simulink model "Hybrid2_article_SVC_stage1"  (R2025a)
settings: Solver=FixedStepAuto  StartTime=0.0  StopTime=0.2  FixedStep=Ts  RelTol=1e-3
undefined symbols (not defined in the file or in its folder): closedLoop, controller, D1, D11, Delta, DiscIntNeverNeededParam, find_system, grid, level, protection, sensor, solarPanel, solarPlant, Ts
libraries: powerlib_extras x38, nesl_utility x29, spsSampleandHoldLib x24, spsThyristorLib x24, spsSeriesRLCBranchLib x23, simulink x22, fl_lib x18, ee_lib x12, spsEdgeDetectorLib x12, spsParallelRLCBranchLib x10, spsThreePhaseVIMeasurementLib x9, simulink_extras x8
(part 3 of 8)

== system Hybrid2_article_SVC_stage1/TSC4 ==
  note: Firing pulses
  note: TSC1
  P : Inport  PortDimensions=6
  Bus to Vector : BusToVector
  Cab : spsSeriesRLCBranchLib/Series RLC Branch  LConnTagsString=__new0  RConnTagsString=__new0  BranchType=RC  Resistance=Rseries  Inductance=1.0  SetiL0=off  InitialCurrent=0  Capacitance=Ccmt  Setx0=off  InitialVoltage=0  Measurements=Branch voltage and current
  Cbc : spsSeriesRLCBranchLib/Series RLC Branch  LConnTagsString=__new0  RConnTagsString=__new0  BranchType=RC  Resistance=Rseries  Inductance=1.0  SetiL0=off  InitialCurrent=0  Capacitance=Ccmt  Setx0=off  InitialVoltage=0  Measurements=None
  Cca : spsSeriesRLCBranchLib/Series RLC Branch  LConnTagsString=__new0  RConnTagsString=__new0  BranchType=RC  Resistance=Rseries  Inductance=1.0  SetiL0=off  InitialCurrent=0  Capacitance=Ccmt  Setx0=off  InitialVoltage=0  Measurements=None
  Demux : Demux  Outputs=6
      settings: DisplayOption=none
  Lab : spsParallelRLCBranchLib/Parallel RLC Branch  LConnTagsString=a  RConnTagsString=__new0  BranchType=RL  Resistance=Rparallel  Inductance=Lcmt  SetiL0=off  InitialCurrent=0  Capacitance=1.0  Setx0=off  InitialVoltage=0  Measurements=None
  Lbc : spsParallelRLCBranchLib/Parallel RLC Branch  LConnTagsString=a  RConnTagsString=__new0  BranchType=RL  Resistance=Rparallel  Inductance=Lcmt  SetiL0=off  InitialCurrent=0  Capacitance=1.0  Setx0=off  InitialVoltage=0  Measurements=None
  Lca : spsParallelRLCBranchLib/Parallel RLC Branch  LConnTagsString=a  RConnTagsString=__new0  BranchType=RL  Resistance=Rparallel  Inductance=Lcmt  SetiL0=off  InitialCurrent=0  Capacitance=1.0  Setx0=off  InitialVoltage=0  Measurements=None
  Selector6 : Selector  InputPortWidth=2  IndexOptions=Index vector (dialog)  Indices=2  OutputSizes=1
  ThAB+ : spsThyristorLib/Thyristor  Ron=Ron  Lon=0  Vf=Vf  IC=0  Rs=Rsnub  Cs=Csnub  Measurements=on
      settings: AttributesFormatString=\n
  ThAB- : spsThyristorLib/Thyristor  Ron=Ron  Lon=0  Vf=Vf  IC=0  Rs=inf  Cs=0  Measurements=off
      settings: AttributesFormatString=\n
  ThBC+ : spsThyristorLib/Thyristor  Ron=Ron  Lon=0  Vf=Vf  IC=0  Rs=Rsnub  Cs=Csnub  Measurements=off
      settings: AttributesFormatString=\n
  ThBC- : spsThyristorLib/Thyristor  Ron=Ron  Lon=0  Vf=Vf  IC=0  Rs=inf  Cs=0  Measurements=off
      settings: AttributesFormatString=\n
  ThCA+ : spsThyristorLib/Thyristor  Ron=Ron  Lon=0  Vf=Vf  IC=0  Rs=Rsnub  Cs=Csnub  Measurements=off
      settings: AttributesFormatString=\n
  ThCA- : spsThyristorLib/Thyristor  Ron=Ron  Lon=0  Vf=Vf  IC=0  Rs=inf  Cs=0  Measurements=off
      settings: AttributesFormatString=\n
  A : PMIOPort  Side=Left
  B : PMIOPort  Port=2  Side=Left
  C : PMIOPort  Port=3  Side=Left
  tag scope: Vth_TSC1ab=global
  wires:
  P/1 -> Demux/1
  [Ap] -> ThAB+/1
  Demux/1 -> [Ap]
  Demux/2 -> [Am]
  Demux/3 -> [Bp]
  Demux/4 -> [Bm]
  Demux/5 -> [Cp]
  [Am] -> ThAB-/1
  [Bp] -> ThBC+/1
  [Bm] -> ThBC-/1
  [Cp] -> ThCA+/1
  [Cm] -> ThCA-/1
  Demux/6 -> [Cm]
  ThAB+/1 -> Bus to Vector/1
  Selector6/1 -> [Vth_TSC1ab]
  Bus to Vector/1 -> Selector6/1
  connections:
  Lab/RConn1 -- Cab/LConn1
  Lab/LConn1 -- ThAB-/LConn1 -- ThAB+/RConn1
  Cca/RConn1 -- A/RConn1 -- ThAB+/LConn1 -- ThAB-/RConn1
  Lbc/LConn1 -- ThBC-/LConn1 -- ThBC+/RConn1
  Cab/RConn1 -- ThBC-/RConn1 -- ThBC+/LConn1 -- B/RConn1
  Lca/LConn1 -- ThCA-/LConn1 -- ThCA+/RConn1
  Cbc/RConn1 -- ThCA-/RConn1 -- ThCA+/LConn1 -- C/RConn1
  Lbc/RConn1 -- Cbc/LConn1
  Lca/RConn1 -- Cca/LConn1

== system Hybrid2_article_SVC_stage1/TSC5 ==
  note: Firing pulses
  P : Inport  PortDimensions=6
  Cab : spsSeriesRLCBranchLib/Series RLC Branch  LConnTagsString=__new0  RConnTagsString=__new0  BranchType=RC  Resistance=Rseries  Inductance=1.0  SetiL0=off  InitialCurrent=0  Capacitance=Ccmt  Setx0=off  InitialVoltage=0  Measurements=Branch voltage and current
  Cbc : spsSeriesRLCBranchLib/Series RLC Branch  LConnTagsString=__new0  RConnTagsString=__new0  BranchType=RC  Resistance=Rseries  Inductance=1.0  SetiL0=off  InitialCurrent=0  Capacitance=Ccmt  Setx0=off  InitialVoltage=0  Measurements=None
  Cca : spsSeriesRLCBranchLib/Series RLC Branch  LConnTagsString=__new0  RConnTagsString=__new0  BranchType=RC  Resistance=Rseries  Inductance=1.0  SetiL0=off  InitialCurrent=0  Capacitance=Ccmt  Setx0=off  InitialVoltage=0  Measurements=None
  Demux : Demux  Outputs=6
      settings: DisplayOption=none
  Lab : spsParallelRLCBranchLib/Parallel RLC Branch  LConnTagsString=a  RConnTagsString=__new0  BranchType=RL  Resistance=Rparallel  Inductance=Lcmt  SetiL0=off  InitialCurrent=0  Capacitance=1.0  Setx0=off  InitialVoltage=0  Measurements=None
  Lbc : spsParallelRLCBranchLib/Parallel RLC Branch  LConnTagsString=a  RConnTagsString=__new0  BranchType=RL  Resistance=Rparallel  Inductance=Lcmt  SetiL0=off  InitialCurrent=0  Capacitance=1.0  Setx0=off  InitialVoltage=0  Measurements=None
  Lca : spsParallelRLCBranchLib/Parallel RLC Branch  LConnTagsString=a  RConnTagsString=__new0  BranchType=RL  Resistance=Rparallel  Inductance=Lcmt  SetiL0=off  InitialCurrent=0  Capacitance=1.0  Setx0=off  InitialVoltage=0  Measurements=None
  ThAB+ : spsThyristorLib/Thyristor  Ron=Ron  Lon=0  Vf=Vf  IC=0  Rs=Rsnub  Cs=Csnub  Measurements=off
      settings: AttributesFormatString=\n
  ThAB- : spsThyristorLib/Thyristor  Ron=Ron  Lon=0  Vf=Vf  IC=0  Rs=inf  Cs=0  Measurements=off
      settings: AttributesFormatString=\n
  ThBC+ : spsThyristorLib/Thyristor  Ron=Ron  Lon=0  Vf=Vf  IC=0  Rs=Rsnub  Cs=Csnub  Measurements=off
      settings: AttributesFormatString=\n
  ThBC- : spsThyristorLib/Thyristor  Ron=Ron  Lon=0  Vf=Vf  IC=0  Rs=inf  Cs=0  Measurements=off
      settings: AttributesFormatString=\n
  ThCA+ : spsThyristorLib/Thyristor  Ron=Ron  Lon=0  Vf=Vf  IC=0  Rs=Rsnub  Cs=Csnub  Measurements=off
      settings: AttributesFormatString=\n
  ThCA- : spsThyristorLib/Thyristor  Ron=Ron  Lon=0  Vf=Vf  IC=0  Rs=inf  Cs=0  Measurements=off
      settings: AttributesFormatString=\n
  A : PMIOPort  Side=Left
  B : PMIOPort  Port=2  Side=Left
  C : PMIOPort  Port=3  Side=Left
  wires:
  Demux/6 -> [Cm]
  [Cm] -> ThCA-/1
  [Cp] -> ThCA+/1
  [Bm] -> ThBC-/1
  [Bp] -> ThBC+/1
  [Am] -> ThAB-/1
  Demux/5 -> [Cp]
  Demux/4 -> [Bm]
  Demux/3 -> [Bp]
  Demux/2 -> [Am]
  Demux/1 -> [Ap]
  [Ap] -> ThAB+/1
  P/1 -> Demux/1
  connections:
  Lca/RConn1 -- Cca/LConn1
  Lbc/RConn1 -- Cbc/LConn1
  C/RConn1 -- ThCA+/LConn1 -- ThCA-/RConn1 -- Cbc/RConn1
  ThCA+/RConn1 -- ThCA-/LConn1 -- Lca/LConn1
  B/RConn1 -- ThBC+/LConn1 -- ThBC-/RConn1 -- Cab/RConn1
  ThBC+/RConn1 -- ThBC-/LConn1 -- Lbc/LConn1
  ThAB-/RConn1 -- ThAB+/LConn1 -- A/RConn1 -- Cca/RConn1
  ThAB+/RConn1 -- ThAB-/LConn1 -- Lab/LConn1
  Lab/RConn1 -- Cab/LConn1

== system Hybrid2_article_SVC_stage1/TSC6 ==
  note: Firing pulses
  P : Inport  PortDimensions=6
  Cab : spsSeriesRLCBranchLib/Series RLC Branch  LConnTagsString=__new0  RConnTagsString=__new0  BranchType=RC  Resistance=Rseries  Inductance=1.0  SetiL0=off  InitialCurrent=0  Capacitance=Ccmt  Setx0=off  InitialVoltage=0  Measurements=Branch voltage and current
  Cbc : spsSeriesRLCBranchLib/Series RLC Branch  LConnTagsString=__new0  RConnTagsString=__new0  BranchType=RC  Resistance=Rseries  Inductance=1.0  SetiL0=off  InitialCurrent=0  Capacitance=Ccmt  Setx0=off  InitialVoltage=0  Measurements=None
  Cca : spsSeriesRLCBranchLib/Series RLC Branch  LConnTagsString=__new0  RConnTagsString=__new0  BranchType=RC  Resistance=Rseries  Inductance=1.0  SetiL0=off  InitialCurrent=0  Capacitance=Ccmt  Setx0=off  InitialVoltage=0  Measurements=None
  Demux : Demux  Outputs=6
      settings: DisplayOption=none
  Lab : spsParallelRLCBranchLib/Parallel RLC Branch  LConnTagsString=a  RConnTagsString=__new0  BranchType=RL  Resistance=Rparallel  Inductance=Lcmt  SetiL0=off  InitialCurrent=0  Capacitance=1.0  Setx0=off  InitialVoltage=0  Measurements=None
  Lbc : spsParallelRLCBranchLib/Parallel RLC Branch  LConnTagsString=a  RConnTagsString=__new0  BranchType=RL  Resistance=Rparallel  Inductance=Lcmt  SetiL0=off  InitialCurrent=0  Capacitance=1.0  Setx0=off  InitialVoltage=0  Measurements=None
  Lca : spsParallelRLCBranchLib/Parallel RLC Branch  LConnTagsString=a  RConnTagsString=__new0  BranchType=RL  Resistance=Rparallel  Inductance=Lcmt  SetiL0=off  InitialCurrent=0  Capacitance=1.0  Setx0=off  InitialVoltage=0  Measurements=None
  ThAB+ : spsThyristorLib/Thyristor  Ron=Ron  Lon=0  Vf=Vf  IC=0  Rs=Rsnub  Cs=Csnub  Measurements=off
      settings: AttributesFormatString=\n
  ThAB- : spsThyristorLib/Thyristor  Ron=Ron  Lon=0  Vf=Vf  IC=0  Rs=inf  Cs=0  Measurements=off
      settings: AttributesFormatString=\n
  ThBC+ : spsThyristorLib/Thyristor  Ron=Ron  Lon=0  Vf=Vf  IC=0  Rs=Rsnub  Cs=Csnub  Measurements=off
      settings: AttributesFormatString=\n
  ThBC- : spsThyristorLib/Thyristor  Ron=Ron  Lon=0  Vf=Vf  IC=0  Rs=inf  Cs=0  Measurements=off
      settings: AttributesFormatString=\n
  ThCA+ : spsThyristorLib/Thyristor  Ron=Ron  Lon=0  Vf=Vf  IC=0  Rs=Rsnub  Cs=Csnub  Measurements=off
      settings: AttributesFormatString=\n
  ThCA- : spsThyristorLib/Thyristor  Ron=Ron  Lon=0  Vf=Vf  IC=0  Rs=inf  Cs=0  Measurements=off
      settings: AttributesFormatString=\n
  A : PMIOPort  Side=Left
  B : PMIOPort  Port=2  Side=Left
  C : PMIOPort  Port=3  Side=Left
  wires:
  P/1 -> Demux/1
  [Ap] -> ThAB+/1
  Demux/1 -> [Ap]
  Demux/2 -> [Am]
  Demux/3 -> [Bp]
  Demux/4 -> [Bm]
  Demux/5 -> [Cp]
  [Am] -> ThAB-/1
  [Bp] -> ThBC+/1
  [Bm] -> ThBC-/1
  [Cp] -> ThCA+/1
  [Cm] -> ThCA-/1
  Demux/6 -> [Cm]
  connections:
  Lab/RConn1 -- Cab/LConn1
  Lab/LConn1 -- ThAB-/LConn1 -- ThAB+/RConn1
  Cca/RConn1 -- A/RConn1 -- ThAB+/LConn1 -- ThAB-/RConn1
  Lbc/LConn1 -- ThBC-/LConn1 -- ThBC+/RConn1
  Cab/RConn1 -- ThBC-/RConn1 -- ThBC+/LConn1 -- B/RConn1
  Lca/LConn1 -- ThCA-/LConn1 -- ThCA+/RConn1
  Cbc/RConn1 -- ThCA-/RConn1 -- ThCA+/LConn1 -- C/RConn1
  Lbc/RConn1 -- Cbc/LConn1
  Lca/RConn1 -- Cca/LConn1

== system Hybrid2_article_SVC_stage1/Variable Load1 ==
  Constant : Constant  Value=[0 -2*pi/3]
  Constant2 : Constant  Value=ModFreq
  Constant3 : Constant  Value=NomPha
  Constant5 : Constant  Value=NomAmp
  Constant6 : Constant  Value=ModAmp
  Demux : Demux  Outputs=2
      settings: DisplayOption=none
  Gain : Gain  Gain=2*pi  SaturateOnIntegerOverflow=on  OutDataTypeStr=Inherit: Same as input  ParamDataTypeStr=Inherit: Same as input
  Ia : spsControlledCurrentSourceLib/Controlled Current Source  Description=source block  Initialize=on  Source_Type=AC  Amplitude=0  Phase=0  Frequency=0  Measurements=None
      settings: AttributesFormatString=\n
  Ib : spsControlledCurrentSourceLib/Controlled Current Source  Description=source block  Initialize=on  Source_Type=AC  Amplitude=0  Phase=0  Frequency=0  Measurements=None
      settings: AttributesFormatString=\n
  Mux : Mux  Inputs=3
  PLL (3ph) : spsPLL3phLib/PLL (3ph)  Fmin=45  Par_Init=[0, 60]  ParK=[60 1400 0]  TcD=3e-2  MaxRateChangeFreq=12  FilterCutOffFreq=25  Ts=Ts  AGC=off
  Product : Product  InputSameDT=on  SaturateOnIntegerOverflow=on  OutDataTypeStr=Inherit: Same as first input
  Product1 : Product  InputSameDT=on  SaturateOnIntegerOverflow=on  OutDataTypeStr=Inherit: Same as first input
  Product2 : Product  Inputs=3  InputSameDT=on  SaturateOnIntegerOverflow=on  OutDataTypeStr=Inherit: Same as first input
  Series RLC Branch1 : spsSeriesRLCBranchLib/Series RLC Branch  LConnTagsString=__new0  RConnTagsString=__new0  BranchType=R  Resistance=1e6  Inductance=1.0  SetiL0=off  InitialCurrent=0  Capacitance=1.0  Setx0=off  InitialVoltage=0  Measurements=None
  Series RLC Branch3 : spsSeriesRLCBranchLib/Series RLC Branch  LConnTagsString=__new0  RConnTagsString=__new0  BranchType=R  Resistance=1e6  Inductance=1.0  SetiL0=off  InitialCurrent=0  Capacitance=1.0  Setx0=off  InitialVoltage=0  Measurements=None
  Sum : Sum  Inputs=+++  InputSameDT=on  SaturateOnIntegerOverflow=on  OutDataTypeStr=Inherit: Same as first input
  Sum1 : Sum  InputSameDT=on  SaturateOnIntegerOverflow=on  OutDataTypeStr=Inherit: Same as first input
  Sum3 : Sum  InputSameDT=on  SaturateOnIntegerOverflow=on  OutDataTypeStr=Inherit: Same as first input
  Terminator1 : Terminator
  Toff : Step  Time=Toff  After=-1  SampleTime=Ts
  Ton : Step  Time=Ton  SampleTime=Ts
  Trigonometric Function : Trigonometry
  Trigonometric Function1 : Trigonometry
  V->pu : Gain  Gain=1/(Vbase*sqrt(2)/sqrt(3))  SaturateOnIntegerOverflow=on  OutDataTypeStr=Inherit: Same as input  ParamDataTypeStr=Inherit: Same as input
  Va : spsVoltageMeasurementLib/Voltage Measurement  Tag=PoWeRsYsTeMmEaSuReMeNt  PhasorSimulation=off  OutputType=Magnitude  PSBequivalent=0
  Va1 : spsVoltageMeasurementLib/Voltage Measurement  Tag=PoWeRsYsTeMmEaSuReMeNt  PhasorSimulation=off  OutputType=Magnitude  PSBequivalent=0
  Va2 : spsVoltageMeasurementLib/Voltage Measurement  Tag=PoWeRsYsTeMmEaSuReMeNt  PhasorSimulation=off  OutputType=Magnitude  PSBequivalent=0
  output Ground1 : spsGroundLib/Ground  LConnTagsString=a  RConnTagsString=__newr0
  t : DigitalClock  SampleTime=Ts
  A : PMIOPort  Side=Left
  B : PMIOPort  Port=2  Side=Left
  C : PMIOPort  Port=3  Side=Left
  wires:
  Sum1/1 -> Product2/1
  Toff/1 -> Sum1/2
  Ton/1 -> Sum1/1
  Constant6/1 -> Product2/2
  Trigonometric Function1/1 -> Product2/3
  Constant5/1 -> Sum3/2
  Product2/1 -> Sum3/1
  Sum3/1 -> Product/2
  Product1/1 -> Trigonometric Function1/1
  t/1 -> Product1/2
  Gain/1 -> Product1/1
  Constant2/1 -> Gain/1
  Constant3/1 -> Sum/3
  Mux/1 -> V->pu/1
  V->pu/1 -> PLL (3ph)/1
  Product/1 -> Demux/1
  Trigonometric Function/1 -> Product/1
  Sum/1 -> Trigonometric Function/1
  Constant/1 -> Sum/2
  Va2/1 -> Mux/3
  Va1/1 -> Mux/2
  Va/1 -> Mux/1
  Demux/1 -> Ia/1
  Demux/2 -> Ib/1
  PLL (3ph)/2 -> Sum/1
  PLL (3ph)/1 -> Terminator1/1
  connections:
  output Ground1/LConn1 -- Va2/LConn2 -- Va1/LConn2 -- Va/LConn2
  Ib/LConn1 -- Series RLC Branch1/LConn1 -- B/RConn1 -- Va1/LConn1
  Ia/LConn1 -- Series RLC Branch3/LConn1 -- A/RConn1 -- Va/LConn1
  Series RLC Branch1/RConn1 -- Series RLC Branch3/RConn1 -- Ia/RConn1 -- Ib/RConn1 -- C/RConn1 -- Va2/LConn1

== system Hybrid2_article_SVC_stage1/Controller/Supply Current to dq ==
  Angle : Inport
  Iabc : Inport  Port=2
  Demux : Demux  Outputs=3
  Filter : TransferFcn  Denominator=[1e-5 1]
  Filter1 : TransferFcn  Denominator=[1e-5 1]
  Park Transform : eeTransforms/Park Transform  AxisAlignment=D-axis  PowerInvariant=off
  Terminator : Terminator
  Id : Outport  VectorParamsAs1DForOutWhenUnconnected=off
  Iq : Outport  Port=2  VectorParamsAs1DForOutWhenUnconnected=off
  wires:
  Demux/1 -> Filter/1
  Park Transform/1 -> Demux/1
  Demux/3 -> Terminator/1
  Filter/1 -> Id/1
  Filter1/1 -> Iq/1
  Demux/2 -> Filter1/1
  Iabc/1 -> Park Transform/1
  Angle/1 -> Park Transform/2

== system Hybrid2_article_SVC_stage1/Controller/Voltage control ==
  e : Inport
  Integrator : Integrator  LimitOutput=on  UpperSaturationLimit=solarPlant.maxPowerACCurrent*sqrt(2)*3/2*1.3  LowerSaturationLimit=-solarPlant.maxPowerACCurrent*sqrt(2)*3/2*1.3
  Ki : Gain  Gain=1/controller.voltagePole
  Kp : Gain  Gain=controller.voltageGain
  Saturation : Saturate  UpperLimit=solarPlant.maxPowerACCurrent*sqrt(2)*3/2*1.3  LowerLimit=-1*solarPlant.maxPowerACCurrent*sqrt(2)*3/2*1.3
  Sum7 : Sum  Inputs=|++
  u : Outport  VectorParamsAs1DForOutWhenUnconnected=off
  wires:
  Integrator/1 -> Sum7/2
  Saturation/1 -> u/1
  Sum7/1 -> Saturation/1
  e/1 -> Kp/1
  Kp/1 -> Ki/1, Sum7/1
  Ki/1 -> Integrator/1

== system Hybrid2_article_SVC_stage1/Controller/d-axis current control ==
  e : Inport
  Integrator : Integrator  LimitOutput=on  UpperSaturationLimit=controller.currentVoltMax  LowerSaturationLimit=-controller.currentVoltMax
  Ki : Gain  Gain=1/controller.currentPole
  Kp : Gain  Gain=controller.currentGain
  Saturation : Saturate  UpperLimit=controller.currentVoltMax  LowerLimit=-1*controller.currentVoltMax
  Sum7 : Sum  Inputs=|++
  u : Outport  VectorParamsAs1DForOutWhenUnconnected=off
  wires:
  Integrator/1 -> Sum7/2
  Saturation/1 -> u/1
  Sum7/1 -> Saturation/1
  e/1 -> Kp/1
  Kp/1 -> Ki/1, Sum7/1
  Ki/1 -> Integrator/1

== system Hybrid2_article_SVC_stage1/Controller/q-axis current control ==
  e : Inport
  Integrator : Integrator  LimitOutput=on  UpperSaturationLimit=controller.currentVoltMax  LowerSaturationLimit=-controller.currentVoltMax
  Ki : Gain  Gain=1/controller.currentPole
  Kp : Gain  Gain=controller.currentGain
  Saturation : Saturate  UpperLimit=controller.currentVoltMax  LowerLimit=-1*controller.currentVoltMax
  Sum7 : Sum  Inputs=|++
  u : Outport  VectorParamsAs1DForOutWhenUnconnected=off
  wires:
  Ki/1 -> Integrator/1
  Kp/1 -> Sum7/1, Ki/1
  e/1 -> Kp/1
  Sum7/1 -> Saturation/1
  Saturation/1 -> u/1
  Integrator/1 -> Sum7/2

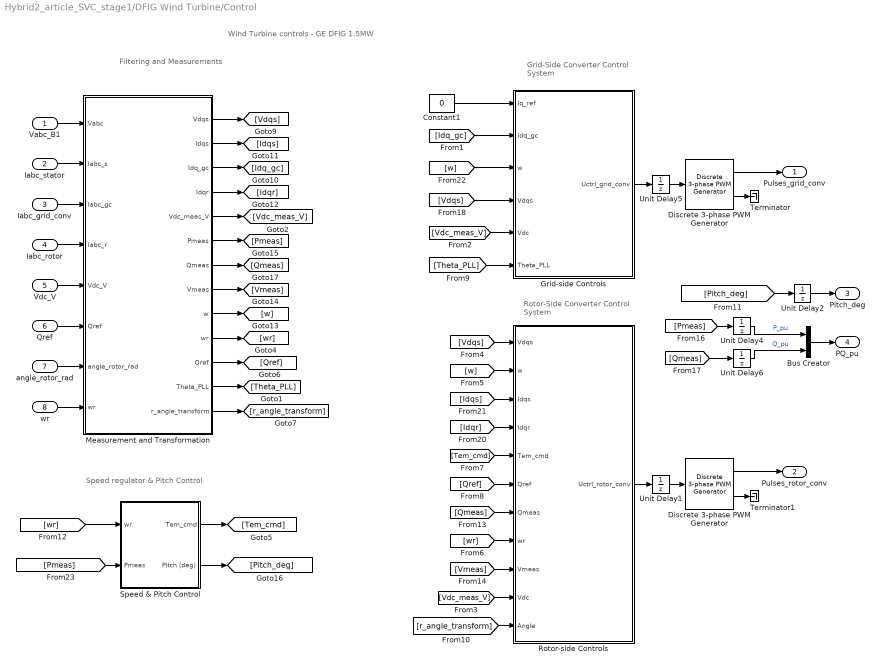
== system Hybrid2_article_SVC_stage1/DFIG Wind Turbine/Control ==
  note: Speed regulator & Pitch Control
  note: Grid-Side Converter
      | Control System
  note: Rotor-Side Converter
      | Control System
  note: Filtering and
      | Measurements
  note: Wind Turbine controls - GE DFIG 1.5MW
  Vabc_B1 : Inport
  Iabc_stator : Inport  Port=2
  Iabc_grid_conv : Inport  Port=3
  Iabc_rotor : Inport  Port=4
  Vdc_V : Inport  Port=5
  Qref : Inport  Port=6
  angle_rotor_rad : Inport  Port=7
  wr : Inport  Port=8
  Bus Creator : BusCreator  Inputs=2
  Constant1 : Constant  Value=0
  Discrete 3-phase PWM Generator : powerlib_extras/Discrete  Control Blocks/Discrete 3-phase PWM Generator  ModulatorType=2-level  ModulatorMode=Un-synchronized  nF=27  Fc=PWM_freq_grid  ModulatingSignals=off  m=0.2  Freq=60  Phase=0  Ts=Ts
  "Discrete 3-phase PWM Generator " : powerlib_extras/Discrete  Control Blocks/Discrete 3-phase PWM Generator  ModulatorType=2-level  ModulatorMode=Un-synchronized  nF=27  Fc=PWM_freq_rotor  ModulatingSignals=off  m=0.2  Freq=60  Phase=0  Ts=Ts
  Grid-side Controls : Subsystem
  Measurement and Transformation : Subsystem
  Rotor-side Controls : Subsystem
  Speed & Pitch Control : Subsystem
  Terminator : Terminator
  Terminator1 : Terminator
  Unit Delay{1..2,4..6} (5 alike) : UnitDelay  SampleTime=Ts  HasFrameUpgradeWarning=on
  Pulses_grid_conv : Outport  VectorParamsAs1DForOutWhenUnconnected=off
  Pulses_rotor_conv : Outport  Port=2  VectorParamsAs1DForOutWhenUnconnected=off
  Pitch_deg : Outport  Port=3  VectorParamsAs1DForOutWhenUnconnected=off
  PQ_pu : Outport  Port=4  VectorParamsAs1DForOutWhenUnconnected=off
  wires:
  Unit Delay6/1 -> Bus Creator/2  "Q_pu"
  Unit Delay4/1 -> Bus Creator/1  "P_pu"
  Unit Delay2/1 -> Pitch_deg/1
  Unit Delay1/1 -> "Discrete 3-phase PWM Generator "/1
  Unit Delay5/1 -> Discrete 3-phase PWM Generator/1
  "Discrete 3-phase PWM Generator "/2 -> Terminator1/1
  Discrete 3-phase PWM Generator/2 -> Terminator/1
  "Discrete 3-phase PWM Generator "/1 -> Pulses_rotor_conv/1
  Discrete 3-phase PWM Generator/1 -> Pulses_grid_conv/1
  Rotor-side Controls/1(Uctrl_rotor_conv) -> Unit Delay1/1
  Grid-side Controls/1(Uctrl_grid_conv) -> Unit Delay5/1
  [Qmeas] -> Unit Delay6/1
  [Pmeas] -> Unit Delay4/1
  Bus Creator/1 -> PQ_pu/1
  Speed & Pitch Control/1(Tem_cmd) -> [Tem_cmd]
  Speed & Pitch Control/2(Pitch (deg)) -> [Pitch_deg]
  [r_angle_transform] -> Rotor-side Controls/11(Angle)
  [Vdc_meas_V] -> Rotor-side Controls/10(Vdc)
  Measurement and Transformation/13(r_angle_transform) -> [r_angle_transform]
  [Theta_PLL] -> Grid-side Controls/6(Theta_PLL)
  Measurement and Transformation/12(Theta_PLL) -> [Theta_PLL]
  [Vmeas] -> Rotor-side Controls/9(Vmeas)
  Measurement and Transformation/8(Vmeas) -> [Vmeas]
  [Qmeas] -> Rotor-side Controls/7(Qmeas)
  Measurement and Transformation/7(Qmeas) -> [Qmeas]
  Vabc_B1/1 -> Measurement and Transformation/1(Vabc)
  Iabc_grid_conv/1 -> Measurement and Transformation/3(Iabc_gc)
  Iabc_rotor/1 -> Measurement and Transformation/4(Iabc_r)
  Iabc_stator/1 -> Measurement and Transformation/2(Iabc_s)
  angle_rotor_rad/1 -> Measurement and Transformation/7(angle_rotor_rad)
  Constant1/1 -> Grid-side Controls/1(Iq_ref)
  Measurement and Transformation/1(Vdqs) -> [Vdqs]
  Measurement and Transformation/2(Idqs) -> [Idqs]
  Measurement and Transformation/3(Idq_gc) -> [Idq_gc]
  Measurement and Transformation/4(Idqr) -> [Idqr]
  Measurement and Transformation/6(Pmeas) -> [Pmeas]
  Measurement and Transformation/9(w) -> [w]
  [Idq_gc] -> Grid-side Controls/2(Idq_gc)
  [w] -> Grid-side Controls/3(w)
  [Vdqs] -> Grid-side Controls/4(Vdqs)
  [Vdc_meas_V] -> Grid-side Controls/5(Vdc)
  [Vdqs] -> Rotor-side Controls/1(Vdqs)
  [w] -> Rotor-side Controls/2(w)
  [Idqs] -> Rotor-side Controls/3(Idqs)
  [Idqr] -> Rotor-side Controls/4(Idqr)
  [Tem_cmd] -> Rotor-side Controls/5(Tem_cmd)
  [Qref] -> Rotor-side Controls/6(Qref)
  [wr] -> Speed & Pitch Control/1(wr)
  Measurement and Transformation/5(Vdc_meas_V) -> [Vdc_meas_V]
  Measurement and Transformation/10("wr ") -> [wr]
  Measurement and Transformation/11("Qref ") -> [Qref]
  Vdc_V/1 -> Measurement and Transformation/5(Vdc_V)
  Qref/1 -> Measurement and Transformation/6(Qref)
  wr/1 -> Measurement and Transformation/8(wr)
  [Pmeas] -> Speed & Pitch Control/2(Pmeas)
  [Pitch_deg] -> Unit Delay2/1
  [wr] -> Rotor-side Controls/8(wr)

== system Hybrid2_article_SVC_stage1/DFIG Wind Turbine/Drive Train ==
  note: Shaft
  note: Turbine
  note: Wind turbine drive train based on a 2-masse model
  T_wt (pu) : Inport
  Generator speed (pu) : Inport  Port=2
  1_2H_WT : Gain  Gain=1/(2*H_WT)  SaturateOnIntegerOverflow=on  OutDataTypeStr=Inherit: Same as input  ParamDataTypeStr=Inherit: Same as input
  Discrete-Time Integrator : DiscreteIntegrator  InitialCondition=w_wt0  SampleTime=Ts  ICPrevOutput=DiscIntNeverNeededParam  ICPrevScaledInput=DiscIntNeverNeededParam
  Discrete-Time Integrator1 : DiscreteIntegrator  InitialCondition=torque0/Ksh  SampleTime=Ts  ICPrevOutput=DiscIntNeverNeededParam  ICPrevScaledInput=DiscIntNeverNeededParam
  Mutual damping : Gain  Gain=D_mutual  SaturateOnIntegerOverflow=on  OutDataTypeStr=Inherit: Same as input  ParamDataTypeStr=Inherit: Same as input
  Stiffness : Gain  Gain=Ksh  SaturateOnIntegerOverflow=on  OutDataTypeStr=Inherit: Same as input  ParamDataTypeStr=Inherit: Same as input
  Sum : Sum  Inputs=+-  InputSameDT=on  SaturateOnIntegerOverflow=on  OutDataTypeStr=Inherit: Same as first input
  Sum1 : Sum  Inputs=+-  InputSameDT=on  SaturateOnIntegerOverflow=on  OutDataTypeStr=Inherit: Same as first input
  Sum2 : Sum  InputSameDT=on  SaturateOnIntegerOverflow=on  OutDataTypeStr=Inherit: Same as first input
  wbase : Gain  Gain=wbase  SaturateOnIntegerOverflow=on  OutDataTypeStr=Inherit: Same as input  ParamDataTypeStr=Inherit: Same as input
  W_wt (pu) : Outport  VectorParamsAs1DForOutWhenUnconnected=off
  T_shaft (pu) : Outport  Port=2  VectorParamsAs1DForOutWhenUnconnected=off
  wires:
  wbase/1 -> Discrete-Time Integrator1/1
  Discrete-Time Integrator1/1 -> Stiffness/1
  Stiffness/1 -> Sum2/1
  Sum/1 -> 1_2H_WT/1
  1_2H_WT/1 -> Discrete-Time Integrator/1
  Discrete-Time Integrator/1 -> Sum1/1, W_wt (pu)/1
  Generator speed (pu)/1 -> Sum1/2
  Sum1/1 -> wbase/1, Mutual damping/1
  Mutual damping/1 -> Sum2/2
  Sum2/1 -> Sum/2, T_shaft (pu)/1
  T_wt (pu)/1 -> Sum/1

== system Hybrid2_article_SVC_stage1/DFIG Wind Turbine/Wind Turbine ==
  W_wt (pu) : Inport
  Pitch angle (deg) : Inport  Port=2
  Wind speed (m/s) : Inport  Port=3
  ->pu : Gain  Gain=1/Prated
  Avoid div. by zero : Saturate  UpperLimit=inf  LowerLimit=eps
  "Avoid div. by zero " : Saturate  UpperLimit=inf  LowerLimit=eps
  Fcn1 : Fcn  Expr=K1*u[2]/u[1]
  Fcn2 : Fcn  Expr=c1*(c6*u[1] + (-c4 - c3*(2.5 + u[2]) + c2*(1/(u[1] + c7*(2.5 + u[2])) -c8/(1 + (2.5 + u[2])^3)))/exp(c5*(1/(u[1] + c7*(2.5 + u[2])) - c8/(1 + (2.5 + u[2])^3))))
  "K2*Cp*wind^3 " : Fcn  Expr=K2*u[1]^3*u[2]
  Mux : Mux  Inputs=2
  Mux1 : Mux  Inputs=2
  Mux2 : Mux  Inputs=2
  Product2 : Product  Inputs=*/  InputSameDT=on  SaturateOnIntegerOverflow=on  OutDataTypeStr=Inherit: Same as first input
  Tt (pu) : Outport  VectorParamsAs1DForOutWhenUnconnected=off
  wires:
  "K2*Cp*wind^3 "/1 -> ->pu/1
  "Avoid div. by zero "/1 -> Product2/2, Mux/2
  Avoid div. by zero/1 -> Mux/1, Mux2/1
  W_wt (pu)/1 -> "Avoid div. by zero "/1
  Pitch angle (deg)/1 -> Mux1/2
  Mux2/1 -> "K2*Cp*wind^3 "/1
  Fcn2/1 -> Mux2/2  "Cp"
  Mux/1 -> Fcn1/1
  Mux1/1 -> Fcn2/1
  Fcn1/1 -> Mux1/1  "lambda"
  Wind speed (m/s)/1 -> Avoid div. by zero/1
  Product2/1 -> Tt (pu)/1
  ->pu/1 -> Product2/1  "power_pu"

== system Hybrid2_article_SVC_stage1/Distribution Statcom1/D_statcom_avg Controller ==
  Vdc : Inport  PortDimensions=1
  Vabc : Inport  Port=2  PortDimensions=3
  Iabc : Inport  Port=3  PortDimensions=3
  Anti-aliasing Filters (7) : Subsystem  mask(Anti-aliasing (2nd order lowpass)){Fc=2000, Ts=Ts}
      mask prompts: Fc "Cut-off frequency (Hz):"; Ts "Sample time:"
  Controller (sample time=Ts*32) : Subsystem
  Unit Delay : UnitDelay  SampleTime=Ts*4  HasFrameUpgradeWarning=on
  Unit Delay1 : UnitDelay  SampleTime=Ts*4  HasFrameUpgradeWarning=on
  Zero-Order Hold1 : ZeroOrderHold  SampleTime=Ts*4
  Zero-Order Hold2 : ZeroOrderHold  SampleTime=Ts*4
  Zero-Order Hold3 : ZeroOrderHold  SampleTime=Ts*4
  m_Phi->Vabc(t) : Subsystem
  w->theta : Subsystem
  Vref_abc : Outport  VectorParamsAs1DForOutWhenUnconnected=off
  wires:
  m_Phi->Vabc(t)/1(Vabc (t)) -> Vref_abc/1
  w->theta/1(theta) -> m_Phi->Vabc(t)/2(theta)
  Unit Delay1/1 -> w->theta/1(w)
  Controller (sample time=Ts*32)/2(w) -> Unit Delay1/1
  Unit Delay/1 -> m_Phi->Vabc(t)/1(m_Phi)
  Controller (sample time=Ts*32)/1(m_Phi) -> Unit Delay/1
  Zero-Order Hold3/1 -> Controller (sample time=Ts*32)/3(Vdc)
  Zero-Order Hold1/1 -> Controller (sample time=Ts*32)/2(Iabc)
  Zero-Order Hold2/1 -> Controller (sample time=Ts*32)/1(Vabc)
  Vdc/1 -> Anti-aliasing Filters (7)/3("Vdc ")
  Iabc/1 -> Anti-aliasing Filters (7)/2("Iabc ")
  Vabc/1 -> Anti-aliasing Filters (7)/1(Vabc)
  Anti-aliasing Filters (7)/3(" Vdc") -> Zero-Order Hold3/1
  Anti-aliasing Filters (7)/2(Iabc) -> Zero-Order Hold1/1
  Anti-aliasing Filters (7)/1(" Vabc") -> Zero-Order Hold2/1

== system Hybrid2_article_SVC_stage1/Filter & AC Measurements/Current Sensor Dynamics ==
  Iabc1 : Inport
  Demux : Demux  Outputs=3
  Mux : Mux  Inputs=3
  Sensor dynamics2 : TransferFcn  Numerator=1  Denominator=[1/sensor.samplingFreq 1]
  Sensor dynamics3 : TransferFcn  Numerator=1  Denominator=[1/sensor.samplingFreq 1]
  Sensor dynamics4 : TransferFcn  Numerator=1  Denominator=[1/sensor.samplingFreq 1]
  Iabc2 : Outport
  tag scope: Ia=global
  wires:
  Iabc1/1 -> Demux/1
  Sensor dynamics3/1 -> Mux/2
  Mux/1 -> Iabc2/1
  Sensor dynamics2/1 -> [Ia], Mux/1
  Demux/1 -> Sensor dynamics2/1
  Demux/3 -> Sensor dynamics4/1
  Demux/2 -> Sensor dynamics3/1
  Sensor dynamics4/1 -> Mux/3

== system Hybrid2_article_SVC_stage1/Filter & AC Measurements/Voltage Sensor Dynamics ==
  Vabc1 : Inport
  Demux : Demux  Outputs=3
  Mux : Mux  Inputs=3
  Sensor dynamics2 : TransferFcn  Numerator=1  Denominator=[1/sensor.samplingFreq 1]
  Sensor dynamics3 : TransferFcn  Numerator=1  Denominator=[1/sensor.samplingFreq 1]
  Sensor dynamics4 : TransferFcn  Numerator=1  Denominator=[1/sensor.samplingFreq 1]
  Vabc2 : Outport
  tag scope: Van=global
  wires:
  Vabc1/1 -> Demux/1
  Sensor dynamics3/1 -> Mux/2
  Mux/1 -> Vabc2/1
  Sensor dynamics2/1 -> [Van], Mux/1
  Demux/1 -> Sensor dynamics2/1
  Demux/3 -> Sensor dynamics4/1
  Demux/2 -> Sensor dynamics3/1
  Sensor dynamics4/1 -> Mux/3

== system Hybrid2_article_SVC_stage1/MPPT/MPPT Algorithm ==
  Ipv : Inport
  Vpv : Inport  Port=2
  IncrementalConductance : Subsystem  VariantControl=false
  PerturbationAndObsrvation : Subsystem  VariantControl=true
  Vmpp : Outport  VectorParamsAs1DForOutWhenUnconnected=off

== system Hybrid2_article_SVC_stage1/Modulation Signal/Gating Signal ==
  Vmod : Inport
  Vdc : Inport  Port=2
  Normalize by DC voltage and disable if DC volts too low : Subsystem
  "[-1,1]" : Saturate  UpperLimit=1  LowerLimit=-1
  mabc : Outport  VectorParamsAs1DForOutWhenUnconnected=off
  wires:
  Normalize by DC voltage and disable if DC volts too low/1(y) -> "[-1,1]"/1
  Vdc/1 -> Normalize by DC voltage and disable if DC volts too low/2(v_dc)
  Vmod/1 -> Normalize by DC voltage and disable if DC volts too low/1(u)
  "[-1,1]"/1 -> mabc/1

== system Hybrid2_article_SVC_stage1/Modulation Signal/dq to alpha beta  ==
  "d " : Inport
  q : Inport  Port=2
  angle : Inport  Port=3
  Constant : Constant  Value=0
  Inverse Park Transform : eeTransforms/Inverse Park Transform  AxisAlignment=D-axis  PowerInvariant=off
  Mux : Mux  Inputs=3
  Vabc : Outport  VectorParamsAs1DForOutWhenUnconnected=off
  wires:
  Inverse Park Transform/1 -> Vabc/1
  angle/1 -> Inverse Park Transform/2
  Mux/1 -> Inverse Park Transform/1
  Constant/1 -> Mux/3
  q/1 -> Mux/2
  "d "/1 -> Mux/1

== system Hybrid2_article_SVC_stage1/PLL and Protection/Protection ==
  w : Inport
  Vsd : Inport  Port=2
  Vpv : Inport  Port=3
  Iac : Inport  Port=4
  AND : Logic  IconShape=distinctive  AllPortsSameDT=off  OutDataTypeStr=boolean
  Constant : Constant  Value=protection.enableTripSignal
  Constant2 : Constant  Value=0
  DC Bus Voltage : Subsystem
  Data Type Conversion : DataTypeConversion  SaturateOnIntegerOverflow=off  RndMeth=Floor
  Grid Frequency : Subsystem
  Grid Over Current : Subsystem
  Grid Voltage : Subsystem
  OR3 : Logic  Operator=OR  Inputs=5  IconShape=distinctive  AllPortsSameDT=off  OutDataTypeStr=boolean
  S-R Flip-Flop : simulink_extras/Flip Flops/S-R Flip-Flop  initial_condition=0
  Short Circuit Current : Subsystem
  Terminator : Terminator
  TS : Outport  VectorParamsAs1DForOutWhenUnconnected=off
  wires:
  Iac/1 -> Grid Over Current/1(Iac), Short Circuit Current/1(Iac)
  Vsd/1 -> Grid Voltage/1(Vsd)
  Grid Voltage/1(Tripsig) -> OR3/1  "GV"
  w/1 -> Grid Frequency/1(w)
  Grid Frequency/1(TripSig) -> OR3/2  "GF"
  Vpv/1 -> DC Bus Voltage/1(Vpv)
  DC Bus Voltage/1(TripSig) -> OR3/3  "DCV"
  Grid Over Current/1(TripSig) -> OR3/4  "GOI"
  Short Circuit Current/1(TripSig) -> OR3/5  "GSC"
  Constant/1 -> AND/2
  AND/1 -> TS/1  "TripSig"
  OR3/1 -> S-R Flip-Flop/1
  S-R Flip-Flop/1 -> AND/1
  Data Type Conversion/1 -> S-R Flip-Flop/2
  Constant2/1 -> Data Type Conversion/1
  S-R Flip-Flop/2 -> Terminator/1

== system Hybrid2_article_SVC_stage1/Power Circuit/DC Current Sensor ==
  Current Sensor : fl_lib/Electrical/Electrical Sensors/Current Sensor
      settings: LogSimulationData=on
  PS-Simulink Converter : nesl_utility/PS-Simulink Converter  PhysicalDomain=network_engine_domain  SubClassName=ps_output  LeftPortType=input  RightPortType=output  PseudoPeriodic=off  Frequencies=[]  VectorFormat=1-D array  Unit=1  AffineConversion=off
  Sensor dynamics : TransferFcn  Numerator=1  Denominator=[1/sensor.samplingFreq 1]
  - : PMIOPort  Side=Left
  + : PMIOPort  Port=2  Side=Right
  tag scope: Ipv=global
  wires:
  PS-Simulink Converter/1 -> Sensor dynamics/1
  Sensor dynamics/1 -> [Ipv]
  connections:
  Current Sensor/RConn2 -- -/RConn1
  +/RConn1 -- Current Sensor/LConn1
  Current Sensor/RConn1 -- PS-Simulink Converter/LConn1

== system Hybrid2_article_SVC_stage1/Power Circuit/DC Voltage Sensor ==
  PS-Simulink Converter : nesl_utility/PS-Simulink Converter  PhysicalDomain=network_engine_domain  SubClassName=ps_output  LeftPortType=input  RightPortType=output  PseudoPeriodic=off  Frequencies=[]  VectorFormat=1-D array  Unit=1  AffineConversion=off
  Sensor dynamics : TransferFcn  Numerator=1  Denominator=[1/sensor.samplingFreq 1]
  Voltage Sensor : fl_lib/Electrical/Electrical Sensors/Voltage Sensor
      settings: LogSimulationData=on
  - : PMIOPort  Side=Left
  + : PMIOPort  Port=2  Side=Right
  tag scope: Vpv=global
  wires:
  PS-Simulink Converter/1 -> Sensor dynamics/1
  Sensor dynamics/1 -> [Vpv]
  connections:
  Voltage Sensor/LConn1 -- +/RConn1
  Voltage Sensor/RConn1 -- PS-Simulink Converter/LConn1
  Voltage Sensor/RConn2 -- -/RConn1

== system Hybrid2_article_SVC_stage1/Power Circuit/Power Circuit ==
  m : Inport
  TripSig : Inport  Port=2
  Average : Subsystem  VariantControl=true
  Three Level : Subsystem  VariantControl=false
  Two Level : Subsystem  VariantControl=false
  + : PMIOPort  Side=Left
  O : PMIOPort  Port=2  Side=Left
  - : PMIOPort  Port=3  Side=Left
  ABC : PMIOPort  Port=4  Side=Right

== system Hybrid2_article_SVC_stage1/SVC Controller1/3-phase signal generator ==
  Constant1 : Constant  Value=60
  Constant2 : Constant  Value=0.9998
  Constant3 : Constant  Value=-2
  Terminator : Terminator
  Three-Phase Sine Generator : spsThreePhaseSineGeneratorLib/Three-Phase Sine Generator  Ts=Ts
  abc : Outport  VectorParamsAs1DForOutWhenUnconnected=off
  wires:
  Constant1/1 -> Three-Phase Sine Generator/3
  Constant2/1 -> Three-Phase Sine Generator/1
  Constant3/1 -> Three-Phase Sine Generator/2
  Three-Phase Sine Generator/1 -> abc/1
  Three-Phase Sine Generator/2 -> Terminator/1

== system Hybrid2_article_SVC_stage1/SVC Controller1/Distribution Unit ==
  note: Bsec = ( 2 - Alpha/90 + sin(2*Alpha)/PI ) * Bsec_nom
  Bsvc : Inport  PortDimensions=1
  Bprim-->Bsec : Fcn  Expr=u[1]/(1 + u[1]*Xf_xfo*100e6/Pnom_xfo)
  Bsec --> Alpha : Lookup_n-D  NumberOfTableDimensions=1  BreakpointsForDimension1=B  BreakpointsForDimension2=[0 571.55 685.8 800.15 914.4 1028.8 1143.1 1257.4 1371.7 1486 1600.3 1714.6 1828.9 1943.2 2057.5 2171.8 2286.1 2400.5 2514.7 2629.1 2743.3 2857.7 2971.9 3086.3 3200.5 3314.9 3429.2]  Table=A  InternalRulePriority=Speed  RndMeth=Simplest
  Data Type Conversion : DataTypeConversion  OutDataTypeStr=boolean  SaturateOnIntegerOverflow=off  RndMeth=Floor
  Data Type Conversion1 : DataTypeConversion  OutDataTypeStr=boolean  SaturateOnIntegerOverflow=off  RndMeth=Floor
  Data Type Conversion2 : DataTypeConversion  OutDataTypeStr=boolean  SaturateOnIntegerOverflow=off  RndMeth=Floor
  Saturation : Saturate  UpperLimit=0  LowerLimit=Bpu_TCR
  Sum1 : Sum  Inputs=+---  InputSameDT=on  SaturateOnIntegerOverflow=on  OutDataTypeStr=Inherit: Same as first input
  TSC1 : Relay  OnSwitchValue=0  OffSwitchValue=-1 * hyst_svc
  TSC1+TSC2 : Relay  OnSwitchValue=0+ Bpu_TSC  OffSwitchValue=-1 * hyst_svc + Bpu_TSC
  TSC1+TSC2+TSC3 : Relay  OnSwitchValue=0+ 2*Bpu_TSC  OffSwitchValue=-1 * hyst_svc + 2*Bpu_TSC
  pu100_puLnom : Gain  Gain=-1/Bpu_TCR  SaturateOnIntegerOverflow=on  OutDataTypeStr=Inherit: Same as input  ParamDataTypeStr=Inherit: Same as input
  pu100_puLnom1 : Gain  Gain=Bpu_TSC  SaturateOnIntegerOverflow=on  OutDataTypeStr=Inherit: Same as input  ParamDataTypeStr=Inherit: Same as input
  pu100_puLnom2 : Gain  Gain=Bpu_TSC  SaturateOnIntegerOverflow=on  OutDataTypeStr=Inherit: Same as input  ParamDataTypeStr=Inherit: Same as input
  pu100_puLnom3 : Gain  Gain=Bpu_TSC  SaturateOnIntegerOverflow=on  OutDataTypeStr=Inherit: Same as input  ParamDataTypeStr=Inherit: Same as input
  Alpha : Outport  InitialOutput=0  VectorParamsAs1DForOutWhenUnconnected=off
  TSC1_On : Outport  Port=2  InitialOutput=0  VectorParamsAs1DForOutWhenUnconnected=off
  TSC2_On : Outport  Port=3  InitialOutput=0  VectorParamsAs1DForOutWhenUnconnected=off
  TSC3_On : Outport  Port=4  InitialOutput=0  VectorParamsAs1DForOutWhenUnconnected=off
  wires:
  pu100_puLnom/1 -> Bsec --> Alpha/1
  Bsec --> Alpha/1 -> Alpha/1
  Bsvc/1 -> Bprim-->Bsec/1
  Bprim-->Bsec/1 -> TSC1+TSC2+TSC3/1, TSC1+TSC2/1, TSC1/1, Sum1/1
  Saturation/1 -> pu100_puLnom/1
  Sum1/1 -> Saturation/1
  pu100_puLnom2/1 -> Sum1/3
  pu100_puLnom3/1 -> Sum1/2
  TSC1/1 -> Data Type Conversion/1, pu100_puLnom3/1
  TSC1+TSC2/1 -> Data Type Conversion1/1, pu100_puLnom2/1
  pu100_puLnom1/1 -> Sum1/4
  TSC1+TSC2+TSC3/1 -> Data Type Conversion2/1, pu100_puLnom1/1
  Data Type Conversion/1 -> TSC1_On/1
  Data Type Conversion1/1 -> TSC2_On/1
  Data Type Conversion2/1 -> TSC3_On/1

== system Hybrid2_article_SVC_stage1/SVC Controller1/Firing Unit ==
  Vabc : Inport  PortDimensions=3
  Alpha : Inport  Port=2  PortDimensions=1
  TSC1_On : Inport  Port=3  OutDataTypeStr=boolean  PortDimensions=1
  TSC2_On : Inport  Port=4  OutDataTypeStr=boolean  PortDimensions=1
  TSC3_On : Inport  Port=5  OutDataTypeStr=boolean  PortDimensions=1
  Demux : Demux  Outputs=3
      settings: DisplayOption=none
  Firing Unit AB : Subsystem  mask{FiringMode=FiringMode, Nstep=Nstep, ParInit=[PhaseInit FreqInit], Ts=Ts}
      mask prompts: FiringMode "Firing Mode (1=Synchronized, 2=Continuous)"; Nstep "Total delay (in number of time step)"; ParInit "Initial phase and frequency of input: [ Phase (degree)  Freq (Hz) ]"; Ts "Sample time:"
      mask init:
      | PhaseInit=ParInit(1);
      | FreqInit=ParInit(2);
  Firing Unit BC : Subsystem  mask{FiringMode=FiringMode, Nstep=Nstep, ParInit=[PhaseInit-120  FreqInit], Ts=Ts}
      mask prompts: FiringMode "Firing Mode (1=Synchronized, 2=Continuous)"; Nstep "Total delay (in number of time step)"; ParInit "Initial phase and frequency of input: [ Phase (degree)  Freq (Hz) ]"; Ts "Sample time:"
      mask init:
      | PhaseInit=ParInit(1);
      | FreqInit=ParInit(2);
  Firing Unit CA : Subsystem  mask{FiringMode=FiringMode, Nstep=Nstep, ParInit=[PhaseInit+120  FreqInit], Ts=Ts}
      mask prompts: FiringMode "Firing Mode (1=Synchronized, 2=Continuous)"; Nstep "Total delay (in number of time step)"; ParInit "Initial phase and frequency of input: [ Phase (degree)  Freq (Hz) ]"; Ts "Sample time:"
      mask init:
      | PhaseInit=ParInit(1);
      | FreqInit=ParInit(2);
  Mux{,1..3} (4 alike) : Mux  Inputs=6
  V->pu : Gain  Gain=1/sqrt(3)  SaturateOnIntegerOverflow=on  OutDataTypeStr=Inherit: Same as input  ParamDataTypeStr=Inherit: Same as input
  TCR_Pulses : Outport  VectorParamsAs1DForOutWhenUnconnected=off
  TSC1_Pulses : Outport  Port=2  VectorParamsAs1DForOutWhenUnconnected=off
  TSC2_Pulses : Outport  Port=3  VectorParamsAs1DForOutWhenUnconnected=off
  TSC3_Pulses : Outport  Port=4  VectorParamsAs1DForOutWhenUnconnected=off
  wires:
  V->pu/1 -> Demux/1
  Alpha/1 -> Firing Unit AB/2(Alpha), Firing Unit CA/2(Alpha), Firing Unit BC/2(Alpha)
  TSC1_On/1 -> Firing Unit CA/3(TSC1_On), Firing Unit BC/3(TSC1_On), Firing Unit AB/3(TSC1_On)
  TSC2_On/1 -> Firing Unit CA/4(TSC2_On), Firing Unit BC/4(TSC2_On), Firing Unit AB/4(TSC2_On)
  Demux/1 -> Firing Unit AB/1(V)
  Demux/2 -> Firing Unit BC/1(V)
  Vabc/1 -> V->pu/1
  Demux/3 -> Firing Unit CA/1(V)
  Firing Unit AB/1(TCR +) -> Mux/1
  Firing Unit AB/2(TCR -) -> Mux/2
  Firing Unit BC/3(TSC1 +) -> Mux1/3
  Firing Unit BC/4(TSC1 -) -> Mux1/4
  Firing Unit BC/1(TCR +) -> Mux/3
  Firing Unit BC/2(TCR -) -> Mux/4
  Firing Unit CA/1(TCR +) -> Mux/5
  Firing Unit CA/2(TCR -) -> Mux/6
  Mux/1 -> TCR_Pulses/1
  Firing Unit AB/3(TSC1 +) -> Mux1/1
  Firing Unit AB/4(TSC1 -) -> Mux1/2
  Firing Unit CA/3(TSC1 +) -> Mux1/5
  Firing Unit CA/4(TSC1 -) -> Mux1/6
  Mux1/1 -> TSC1_Pulses/1
  Firing Unit AB/5(TSC2 +) -> Mux2/1
  Firing Unit AB/6(TSC2 -) -> Mux2/2
  Mux2/1 -> TSC2_Pulses/1
  Firing Unit BC/5(TSC2 +) -> Mux2/3
  Firing Unit BC/6(TSC2 -) -> Mux2/4
  Firing Unit CA/5(TSC2 +) -> Mux2/5
  Firing Unit CA/6(TSC2 -) -> Mux2/6
  TSC3_On/1 -> Firing Unit CA/5(TSC3_On), Firing Unit BC/5(TSC3_On), Firing Unit AB/5(TSC3_On)
  Mux3/1 -> TSC3_Pulses/1
  Firing Unit AB/7(TSC3 +) -> Mux3/1
  Firing Unit AB/8(TSC3 -) -> Mux3/2
  Firing Unit BC/7(TSC3 +) -> Mux3/3
  Firing Unit BC/8(TSC3 -) -> Mux3/4
  Firing Unit CA/7(TSC3 +) -> Mux3/5
  Firing Unit CA/8(TSC3 -) -> Mux3/6

== system Hybrid2_article_SVC_stage1/SVC Controller1/Info ==
  note: 1) Open-loop time constant evaluation:
  note: Xs -> Slope in pu/100MVA
      |  Ki -> Integral gain (puB/puV/s)
  note: where:
  note: Closed-loop time constant --> Tc ~= [ Xs / ( Xr + Xs ) ] * To
  note: Open-loop time constant --> To ~= 1 / ( Ki * Xs )
  note: To verify the following formula, open the loop (using the manual switch) and
      | add a 0.008 pu step to the reference voltage (Vref)
  note: 2) Misfiring simulation:
  note: To simulate a misfiring of thyristor AB+ of TSC1:
      | First switch off the TSC1 branch by adding a -0.008 pu to Vref at 0.04s
      | and then generate a firing pulse at 0.105s (one time step duration) using the Timer block

== system Hybrid2_article_SVC_stage1/SVC Controller1/Measurement System ==
  Vabc : Inport  PortDimensions=3
  PLL (3ph) : spsPLL3phLib/PLL (3ph)  Fmin=45  Par_Init=[Phase_Init Freq_Init]  ParK=[60 1400 0]  TcD=3e-2  MaxRateChangeFreq=12  FilterCutOffFreq=25  Ts=Ts  AGC=off
  Positive-Sequence (PLL-Driven) : spsPositiveSequencePLLDrivenLib/Positive-Sequence (PLL-Driven)  Finit=Freq_Init  Fmin=45  InInit=[Mag_Init 0]  Ts=Ts
  Terminator2 : Terminator
  Vmes : Outport  VectorParamsAs1DForOutWhenUnconnected=off
  wires:
  PLL (3ph)/1 -> Positive-Sequence (PLL-Driven)/1
  PLL (3ph)/2 -> Positive-Sequence (PLL-Driven)/2
  Vabc/1 -> Positive-Sequence (PLL-Driven)/3, PLL (3ph)/1
  Positive-Sequence (PLL-Driven)/2 -> Terminator2/1
  Positive-Sequence (PLL-Driven)/1 -> Vmes/1

== system Hybrid2_article_SVC_stage1/SVC Controller1/Voltage Regulator ==
  note: Xs -> Slope in pu/100MVA
      |  Ki -> Integral gain (puB/puV/s)
  note: where:
  note: Closed-loop time constant --> Tc = [ Xs / ( Xr + Xs ) ] * To
  note: Open-loop time constant --> To = 1 / ( Ki * Xs )
  Vmes : Inport  PortDimensions=1
  Bref : Inport  Port=2  PortDimensions=1
  Vref : Inport  Port=3
  Constant : Constant  Value=OpMode
  Constant10 : Constant
  Droop : Gain  Gain=Xs  SaturateOnIntegerOverflow=on  OutDataTypeStr=Inherit: Same as input  ParamDataTypeStr=Inherit: Same as input
  Gain1 : Gain  Gain=Kp  SaturateOnIntegerOverflow=on  OutDataTypeStr=Inherit: Same as input  ParamDataTypeStr=Inherit: Same as input
  Gain2 : Gain  Gain=Ki  SaturateOnIntegerOverflow=on  OutDataTypeStr=Inherit: Same as input  ParamDataTypeStr=Inherit: Same as input
  Integrateur : DiscreteIntegrator  SampleTime=Ts  LimitOutput=on  UpperSaturationLimit=Bmax  LowerSaturationLimit=Bmin  ICPrevOutput=DiscIntNeverNeededParam  ICPrevScaledInput=DiscIntNeverNeededParam
  Prod. : Product  InputSameDT=on  SaturateOnIntegerOverflow=on  OutDataTypeStr=Inherit: Same as first input
  Relational Operator2 : RelationalOperator  Operator=~=
  Som : Sum  Inputs=-+  InputSameDT=on  SaturateOnIntegerOverflow=on  OutDataTypeStr=Inherit: Same as first input
  Som1 : Sum  Inputs=-+  InputSameDT=on  SaturateOnIntegerOverflow=on  OutDataTypeStr=Inherit: Same as first input
  Som2 : Sum  InputSameDT=on  SaturateOnIntegerOverflow=on  OutDataTypeStr=Inherit: Same as first input
  Switch2 : Switch  Criteria=u2 > Threshold
  Unit Delay1 : UnitDelay  SampleTime=Ts  HasFrameUpgradeWarning=on
  Bsvc : Outport  InitialOutput=0  VectorParamsAs1DForOutWhenUnconnected=off
  wires:
  Constant/1 -> Relational Operator2/2
  Som1/1 -> Gain2/1, Gain1/1  "err"
  Gain2/1 -> Integrateur/1
  Relational Operator2/1 -> Switch2/2
  Bref/1 -> Switch2/1
  Som2/1 -> Switch2/3
  Switch2/1 -> Unit Delay1/1, Bsvc/1
  Vmes/1 -> Prod./1, Som/1
  Vref/1 -> Som/2
  Droop/1 -> Som1/1
  Som/1 -> Som1/2
  Constant10/1 -> Relational Operator2/1
  Unit Delay1/1 -> Prod./2
  Integrateur/1 -> Som2/2
  Gain1/1 -> Som2/1
  Prod./1 -> Droop/1

== system Hybrid2_article_SVC_stage1/Solar Plant/Solar Panel ==
  Current-Controlled Current Source : fl_lib/Electrical/Electrical Sources/Current-Controlled Current Source  K=-1*(solarPanel.numParallelCell-1)  i1_specify=off  i1_priority=None  i1=0 A  i1_nominal_specify=off  i1_nominal_value=1  i1_nominal_unit=A  i2_specify=off  i2_priority=None  i2=0 A  i2_nominal_specify=off  i2_nominal_value=1  i2_nominal_unit=A
      settings: InternalSimscapePortConfiguration="{\"Bottom\":[],\"Left\":[{\"id\":\"p1\",\"label\":\"+\",\"type\":\"foundation.electrical.electrical\"},{\"id\":\"head\",\"label\":\"\",\"type\":\"foundation.electrical.electrical\"}],\"Right\":[{\"id\":\"n1\",\"label\":\"-\",\"type\":\"foundation.electrical.electrical\"},{\"id\":\"tail\",\"label\":\"\",\"type\":\"foundation.electrical.electrical\"}],\"Top\":[]}"
  Solar Cell : ee_lib/Sources/Solar Cell  prm=1  Isc=solarPanel.shortCircuitCurrentPV/solarPanel.numParallelCell A  Voc=solarPanel.openCircuitVoltagePV/solarPanel.numSeriesCell V  Is=1e-6 A  Is2=0 A  Iph=7.34 A  Ir0=solarPanel.irradianceMeasurement W/m^2  ec=solarPanel.qualityFactor  N2=2  Rs=solarPanel.seriesResistance Ohm  Rp=inf Ohm  N_series=solarPanel.numSeriesCell-1  N_parallel=1  TIPH1=solarPanel.currentTemperatureCoeff 1/K  EG=1.11 eV  TXIS1=solarPanel.temperatureExponent  TXIS2=3  TRS1=0  TRP1=0  Tmeas=solarPanel.temperatureMeasurement degC  TFIXED=solarPanel.temperature degC  thermal_mass=100 J/K  initial_temperature=25 degC
  Ir : PMIOPort  Side=Left
  + : PMIOPort  Port=2  Side=Right
  - : PMIOPort  Port=3  Side=Right
  connections:
  Current-Controlled Current Source/LConn2 -- -/RConn1 -- Solar Cell/RConn1
  Ir/RConn1 -- Solar Cell/LConn1
  Current-Controlled Current Source/LConn1 -- Solar Cell/LConn2
  Current-Controlled Current Source/RConn1 -- Current-Controlled Current Source/RConn2 -- +/RConn1
